simulink model "body2"  (Simulink 7.5)
settings: Solver=ode45  StartTime=0.0  StopTime=10.0  RelTol=1e-3
settings Model: Creator=ex08148  LastModifiedBy=ex08148

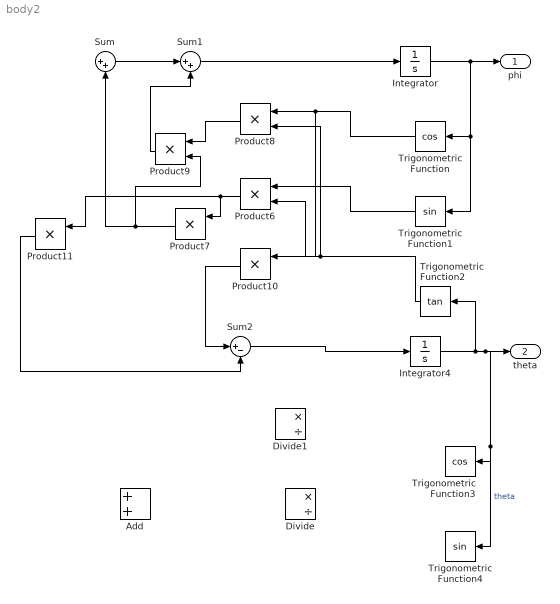
== system body2 ==
  Add : Sum  OutDataType=fixdt(1, 16)  OutScaling=2^-10
  Divide : Product  Inputs=*/  OutDataType=fixdt(1, 16)  OutScaling=2^-10
  Divide1 : Product  Inputs=*/  OutDataType=fixdt(1, 16)  OutScaling=2^-10
  Integrator : Integrator
  Integrator4 : Integrator
  Product{6..11} (6 alike) : Product  OutDataType=fixdt(1, 16)  OutScaling=2^0  RndMeth=Zero
  Sum : Sum  Inputs=|++  OutDataType=fixdt(1, 16)  OutScaling=2^0
  Sum1 : Sum  Inputs=|++  OutDataType=fixdt(1, 16)  OutScaling=2^0
  Sum2 : Sum  Inputs=|+-  OutDataType=fixdt(1, 16)  OutScaling=2^0
  Trigonometric Function : Trigonometry  Operator=cos
  Trigonometric Function1 : Trigonometry
  Trigonometric Function2 : Trigonometry  Operator=tan
  Trigonometric Function3 : Trigonometry  Operator=cos
  Trigonometric Function4 : Trigonometry
  phi : Outport  OutDataType=fixdt(1, 16)  OutScaling=2^0
  theta : Outport  Port=2  OutDataType=fixdt(1, 16)  OutScaling=2^0
  wires:
  Sum/1 -> Sum1/1
  Sum1/1 -> Integrator/1
  Integrator/1 -> phi/1, Trigonometric Function/1, Trigonometric Function1/1
  Trigonometric Function/1 -> Product8/1, Product10/1
  Trigonometric Function1/1 -> Product6/1
  Trigonometric Function2/1 -> Product6/2, Product8/2
  Product10/1 -> Sum2/1
  Sum2/1 -> Integrator4/1
  Integrator4/1 -> Trigonometric Function2/1, theta/1, Trigonometric Function3/1, Trigonometric Function4/1  "theta"
  Product8/1 -> Product9/1
  Product9/1 -> Sum1/2
  Product6/1 -> Product7/1, Product11/1
  Product7/1 -> Sum/2, Product9/2
  Product11/1 -> Sum2/2
